simulink model "amk_eff_estimator_base"  (R2024b)
settings: Solver=FixedStepAuto  StartTime=0.0  StopTime=10.0  FixedStep=0.004  RelTol=1e-3
undefined symbols (not defined in the file): AMKData, AMKData_T100C, AMKData_T120C
settings Model: Creator=lukec  LastModifiedBy=lukec
settings OptimizationCC: DefaultParameterBehavior=Inlined  EnhancedBackFolding=on  PassReuseOutputArgsAs=Individual arguments  ZeroExternalMemoryAtStartup=off  ZeroInternalMemoryAtStartup=off  OptimizeBlockOrder=speed  DifferentSizesBufferReuse=on  OptimizationCustomize=off  EfficientTunableParamExpr=on
settings DebuggingCC: ParameterTunabilityLossMsg=error
settings HardwareCC: ProdBitPerPointer=32  ProdBitPerSizeT=32  ProdBitPerPtrDiffT=32  ProdLargestAtomicInteger=Long  ProdLargestAtomicFloat=Double  ProdWordSize=32  ProdHWDeviceType=ARM Compatible->ARM Cortex-M
settings SFSimCC: MATLABDynamicMemAlloc=off
settings RTWCC: Description=Embedded Coder  SystemTargetFile=ert.tlc  GenCodeOnly=on  PackageGeneratedCodeAndArtifacts=on  TemplateMakefile=ert_default_tmf  Toolchain=CMake  TargetLang=C++  HalideCodeGeneration=on
settings CodeAppCC: ForceParamTrailComments=on  IgnoreCustomStorageClasses=off  MaxIdLength=255  OperatorAnnotations=on  SimulinkDataObjDesc=on  SFDataObjDesc=on  InsertBlockDesc=on
settings ERTTargetCC: TargetLangStandard=C++17 (ISO)  CodeInterfacePackaging=C++ class  RootIOFormat=Structure reference  ERTCustomFileTemplate=example_file_process.tlc  ArrayContainerType=std::array

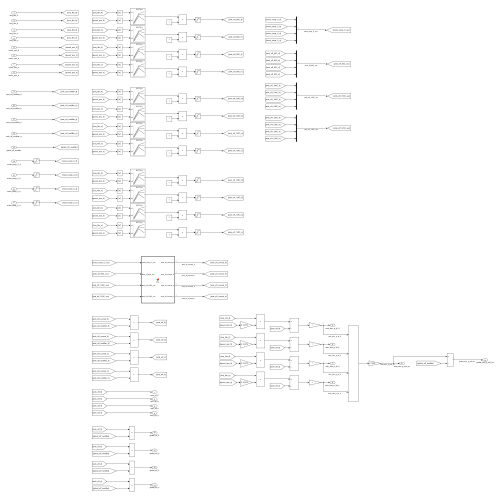
[thumbnail: Simulink's stored preview of the top-level diagram]
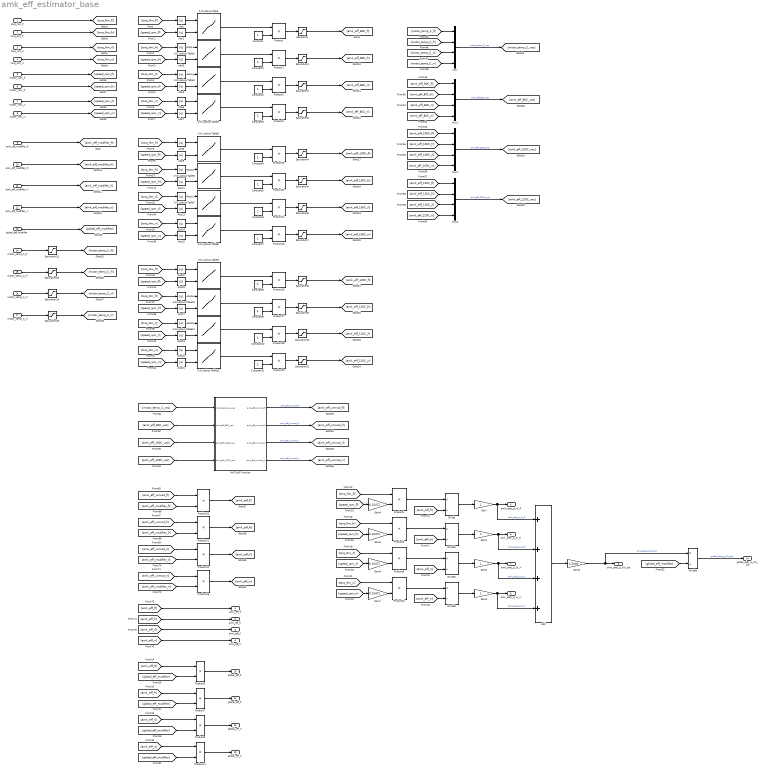
== system amk_eff_estimator_base ==
  torq_Nm_fl : Inport
  torq_Nm_fr : Inport  Port=2
  torq_Nm_rl : Inport  Port=3
  torq_Nm_rr : Inport  Port=4
  motor_rpm_fl : Inport  Port=5
  motor_rpm_fr : Inport  Port=6
  motor_rpm_rl : Inport  Port=7
  motor_rpm_rr : Inport  Port=8
  amk_eff_modifier_fl : Inport  Port=9
  amk_eff_modifier_fr : Inport  Port=10
  amk_eff_modifier_rl : Inport  Port=11
  amk_eff_modifier_rr : Inport  Port=12
  global_eff_modifier : Inport  Port=13
  motor_temp_C_fl : Inport  Port=14
  motor_temp_C_fr : Inport  Port=15
  motor_temp_C_rl : Inport  Port=16
  motor_temp_C_rr : Inport  Port=17
  2-D Lookup Table{,1..3} (4 alike) : Lookup_n-D  BreakpointsForDimension1=AMKData.torq_testpoints  BreakpointsForDimension2=AMKData.speed_testpoints  Table=AMKData.eff_zq  ExtrapMethod=Clip  UseLastTableValue=on  InternalRulePriority=Speed  RndMeth=Simplest
      settings: InputPortMap=u0,u1
  2-D Lookup Table{9..12} (4 alike) : Lookup_n-D  BreakpointsForDimension1=AMKData_T120C.torq_testpoints  BreakpointsForDimension2=AMKData_T120C.speed_testpoints  Table=AMKData_T120C.eff_zq  ExtrapMethod=Clip  UseLastTableValue=on  InternalRulePriority=Speed  RndMeth=Simplest
      settings: InputPortMap=u0,u1
  2-D Lookup Table{5..8} (4 alike) : Lookup_n-D  BreakpointsForDimension1=AMKData_T100C.torq_testpoints  BreakpointsForDimension2=AMKData_T100C.speed_testpoints  Table=AMKData_T100C.eff_zq  ExtrapMethod=Clip  UseLastTableValue=on  InternalRulePriority=Speed  RndMeth=Simplest
      settings: InputPortMap=u0,u1
  Abs{,1..23} (24 alike) : Abs  SaturateOnIntegerOverflow=off
  Add : Sum  Inputs=++++
  Constant{,1..11} (12 alike) : Constant
  Divide{,1..4} (5 alike) : Product  Inputs=*/
  Gain{,1..3} (4 alike) : Gain
  Gain{4..7} (4 alike) : Gain  Gain=0.10472
  Gain8 : Gain  Gain=1/1000
  MATLAB Function : MATLAB Function  TreatAsAtomicUnit=on
  Mux{,1..3} (4 alike) : Mux
  Product{,1..23} (24 alike) : Product
  Saturation{,1..11} (12 alike) : Saturate  UpperLimit=1  LowerLimit=0.6
  Saturation{12..15} (4 alike) : Saturate  UpperLimit=120  LowerLimit=80
  amk_eff_fl : Outport
  amk_eff_fr : Outport  Port=2
  amk_eff_rl : Outport  Port=3
  amk_eff_rr : Outport  Port=4
  amk_elec_p_W_fl : Outport  Port=5
  amk_elec_p_W_fr : Outport  Port=6
  amk_elec_p_W_rl : Outport  Port=7
  amk_elec_p_W_rr : Outport  Port=8
  amk_elec_p_kW_tot : Outport  Port=9
  global_eff_fl : Outport  Port=10
  global_eff_fr : Outport  Port=11
  global_eff_rl : Outport  Port=12
  global_eff_rr : Outport  Port=13
  global_elec_p_kW_tot : Outport  Port=14
  wires:
  torq_Nm_rl/1 -> [torq_Nm_rl]
  Constant2/1 -> Product2/2
  [speed_rpm_fl] -> Abs1/1
  Abs5/1 -> 2-D Lookup Table2/2
  motor_rpm_rr/1 -> [speed_rpm_rr]
  2-D Lookup Table/1 -> Product/1
  Product/1 -> Saturation/1
  [speed_rpm_fr] -> Abs3/1
  motor_rpm_fl/1 -> [speed_rpm_fl]
  Abs/1 -> 2-D Lookup Table/1
  Constant3/1 -> Product3/2
  2-D Lookup Table2/1 -> Product2/1
  Abs7/1 -> 2-D Lookup Table3/2
  [torq_Nm_fr] -> Abs2/1
  Abs2/1 -> 2-D Lookup Table1/1
  Constant/1 -> Product/2
  [torq_Nm_rl] -> Abs4/1
  2-D Lookup Table3/1 -> Product3/1
  torq_Nm_rr/1 -> [torq_Nm_rr]
  2-D Lookup Table1/1 -> Product1/1
  amk_eff_modifier_fl/1 -> [amk_eff_modifier_fl]
  motor_rpm_rl/1 -> [speed_rpm_rl]
  Constant1/1 -> Product1/2
  Abs1/1 -> 2-D Lookup Table/2
  torq_Nm_fl/1 -> [torq_Nm_fl]
  Abs3/1 -> 2-D Lookup Table1/2
  [torq_Nm_fl] -> Abs/1
  [speed_rpm_rl] -> Abs5/1
  Abs6/1 -> 2-D Lookup Table3/1
  motor_rpm_fr/1 -> [speed_rpm_fr]
  [speed_rpm_rr] -> Abs7/1
  Abs4/1 -> 2-D Lookup Table2/1
  [torq_Nm_rr] -> Abs6/1
  torq_Nm_fr/1 -> [torq_Nm_fr]
  [torq_Nm_fl] -> Product4/1
  [speed_rpm_fl] -> Gain4/1
  Product1/1 -> Saturation1/1
  Product2/1 -> Saturation2/1
  Product3/1 -> Saturation3/1
  Product4/1 -> Divide/1
  [amk_eff_fl] -> Divide/2
  Divide/1 -> Gain/1
  Divide1/1 -> Gain1/1
  [amk_eff_fr] -> Divide1/2
  Product6/1 -> Divide1/1
  [speed_rpm_fr] -> Gain5/1
  [torq_Nm_fr] -> Product6/1
  [torq_Nm_rl] -> Product8/1
  [speed_rpm_rl] -> Gain6/1
  Product8/1 -> Divide2/1
  [amk_eff_rl] -> Divide2/2
  Divide2/1 -> Gain2/1
  Divide3/1 -> Gain3/1
  [amk_eff_rr] -> Divide3/2
  Product10/1 -> Divide3/1
  [speed_rpm_rr] -> Gain7/1
  [torq_Nm_rr] -> Product10/1
  Gain/1 -> Add/1, amk_elec_p_W_fl/1  "amk_elec_p_W_fl"
  Gain1/1 -> Add/2, amk_elec_p_W_fr/1  "amk_elec_p_W_fr"
  Gain2/1 -> Add/3, amk_elec_p_W_rl/1  "amk_elec_p_W_rl"
  Gain3/1 -> Add/4, amk_elec_p_W_rr/1  "amk_elec_p_W_rr"
  Gain4/1 -> Product4/2
  Gain5/1 -> Product6/2
  Gain6/1 -> Product8/2
  Gain7/1 -> Product10/2
  Add/1 -> Gain8/1
  Saturation/1 -> [amk_eff_80C_fl]
  Saturation1/1 -> [amk_eff_80C_fr]
  Saturation2/1 -> [amk_eff_80C_rl]
  Saturation3/1 -> [amk_eff_80C_rr]
  amk_eff_modifier_fr/1 -> [amk_eff_modifier_fr]
  amk_eff_modifier_rl/1 -> [amk_eff_modifier_rl]
  amk_eff_modifier_rr/1 -> [amk_eff_modifier_rr]
  global_eff_modifier/1 -> [global_eff_modifier]
  [amk_eff_fl] -> Product5/1
  [global_eff_modifier] -> Product5/2
  Product5/1 -> global_eff_fl/1
  [global_eff_modifier] -> Product7/2
  [amk_eff_fr] -> Product7/1
  Product7/1 -> global_eff_fr/1
  [global_eff_modifier] -> Product9/2
  [amk_eff_rl] -> Product9/1
  Product9/1 -> global_eff_rl/1
  [global_eff_modifier] -> Product11/2
  [amk_eff_rr] -> Product11/1
  Product11/1 -> global_eff_rr/1
  [global_eff_modifier] -> Divide4/2
  Divide4/1 -> global_elec_p_kW_tot/1  "global_elec_p_kW_tot"
  Gain8/1 -> Divide4/1, amk_elec_p_kW_tot/1  "amk_elec_p_kW_tot"
  Product15/1 -> Saturation7/1
  Product14/1 -> Saturation6/1
  Product13/1 -> Saturation5/1
  [torq_Nm_rr] -> Abs14/1
  Abs12/1 -> 2-D Lookup Table7/1
  [speed_rpm_rr] -> Abs15/1
  Abs14/1 -> 2-D Lookup Table8/1
  [speed_rpm_rl] -> Abs13/1
  [torq_Nm_fl] -> Abs8/1
  Abs11/1 -> 2-D Lookup Table6/2
  Abs9/1 -> 2-D Lookup Table5/2
  Constant5/1 -> Product13/2
  2-D Lookup Table6/1 -> Product13/1
  2-D Lookup Table8/1 -> Product15/1
  [torq_Nm_rl] -> Abs12/1
  Constant4/1 -> Product12/2
  Abs10/1 -> 2-D Lookup Table6/1
  [torq_Nm_fr] -> Abs10/1
  Abs15/1 -> 2-D Lookup Table8/2
  2-D Lookup Table7/1 -> Product14/1
  Constant7/1 -> Product15/2
  Abs8/1 -> 2-D Lookup Table5/1
  [speed_rpm_fr] -> Abs11/1
  Product12/1 -> Saturation4/1
  2-D Lookup Table5/1 -> Product12/1
  Abs13/1 -> 2-D Lookup Table7/2
  [speed_rpm_fl] -> Abs9/1
  Constant6/1 -> Product14/2
  Constant10/1 -> Product18/2
  [speed_rpm_fl] -> Abs23/1
  Abs19/1 -> 2-D Lookup Table11/2
  2-D Lookup Table9/1 -> Product16/1
  Product16/1 -> Saturation8/1
  [speed_rpm_fr] -> Abs17/1
  Abs22/1 -> 2-D Lookup Table9/1
  Constant11/1 -> Product19/2
  2-D Lookup Table11/1 -> Product18/1
  Abs21/1 -> 2-D Lookup Table12/2
  [torq_Nm_fr] -> Abs16/1
  Abs16/1 -> 2-D Lookup Table10/1
  Constant8/1 -> Product16/2
  [torq_Nm_rl] -> Abs18/1
  2-D Lookup Table12/1 -> Product19/1
  2-D Lookup Table10/1 -> Product17/1
  Constant9/1 -> Product17/2
  Abs23/1 -> 2-D Lookup Table9/2
  Abs17/1 -> 2-D Lookup Table10/2
  [torq_Nm_fl] -> Abs22/1
  [speed_rpm_rl] -> Abs19/1
  Abs20/1 -> 2-D Lookup Table12/1
  [speed_rpm_rr] -> Abs21/1
  Abs18/1 -> 2-D Lookup Table11/1
  [torq_Nm_rr] -> Abs20/1
  Product17/1 -> Saturation9/1
  Product18/1 -> Saturation10/1
  Product19/1 -> Saturation11/1
  Saturation4/1 -> [amk_eff_100C_fl]
  Saturation5/1 -> [amk_eff_100C_fr]
  Saturation6/1 -> [amk_eff_100C_rl]
  Saturation7/1 -> [amk_eff_100C_rr]
  Saturation8/1 -> [amk_eff_120C_fl]
  Saturation9/1 -> [amk_eff_120C_fr]
  Saturation10/1 -> [amk_eff_120C_rl]
  Saturation11/1 -> [amk_eff_120C_rr]
  motor_temp_C_fl/1 -> Saturation12/1
  motor_temp_C_fr/1 -> Saturation13/1
  motor_temp_C_rl/1 -> Saturation14/1
  motor_temp_C_rr/1 -> Saturation15/1
  Saturation12/1 -> [motor_temp_C_fl]
  Saturation13/1 -> [motor_temp_C_fr]
  Saturation14/1 -> [motor_temp_C_rl]
  Saturation15/1 -> [motor_temp_C_rr]
  [motor_temp_C_fl] -> Mux/1
  [motor_temp_C_fr] -> Mux/2
  [motor_temp_C_rl] -> Mux/3
  [motor_temp_C_rr] -> Mux/4
  Mux/1 -> [motor_temp_C_vec]  "motor_temp_C_vec"
  [amk_eff_80C_fl] -> Mux1/1
  [amk_eff_80C_fr] -> Mux1/2
  [amk_eff_80C_rl] -> Mux1/3
  [amk_eff_80C_rr] -> Mux1/4
  Mux1/1 -> [amk_eff_80C_vec]  "amk_eff_80C_vec"
  Mux2/1 -> [amk_eff_100C_vec]  "amk_eff_100C_vec"
  [amk_eff_100C_rr] -> Mux2/4
  [amk_eff_100C_rl] -> Mux2/3
  [amk_eff_100C_fr] -> Mux2/2
  [amk_eff_100C_fl] -> Mux2/1
  [amk_eff_120C_fl] -> Mux3/1
  [amk_eff_120C_fr] -> Mux3/2
  [amk_eff_120C_rl] -> Mux3/3
  [amk_eff_120C_rr] -> Mux3/4
  Mux3/1 -> [amk_eff_120C_vec]  "amk_eff_120C_vec"
  [motor_temp_C_vec] -> MATLAB Function/1(motor_temp_C_vec)
  [amk_eff_80C_vec] -> MATLAB Function/2(amk_eff_80C_vec)
  [amk_eff_100C_vec] -> MATLAB Function/3(amk_eff_100C_vec)
  [amk_eff_120C_vec] -> MATLAB Function/4(amk_eff_120C_vec)
  MATLAB Function/1(amk_eff_unmod_fl) -> [amk_eff_unmod_fl]  "amk_eff_unmod_fl"
  MATLAB Function/2(amk_eff_unmod_fr) -> [amk_eff_unmod_fr]  "amk_eff_unmod_fr"
  MATLAB Function/3(amk_eff_unmod_rl) -> [amk_eff_unmod_rl]  "amk_eff_unmod_rl"
  MATLAB Function/4(amk_eff_unmod_rr) -> [amk_eff_unmod_rr]  "amk_eff_unmod_rr"
  [amk_eff_unmod_fl] -> Product20/1
  [amk_eff_modifier_fl] -> Product20/2
  Product20/1 -> [amk_eff_fl]
  Product21/1 -> [amk_eff_fr]
  [amk_eff_modifier_fr] -> Product21/2
  [amk_eff_unmod_fr] -> Product21/1
  [amk_eff_unmod_rl] -> Product22/1
  [amk_eff_modifier_rl] -> Product22/2
  Product22/1 -> [amk_eff_rl]
  Product23/1 -> [amk_eff_rr]
  [amk_eff_modifier_rr] -> Product23/2
  [amk_eff_unmod_rr] -> Product23/1
  [amk_eff_fl] -> amk_eff_fl/1
  [amk_eff_fr] -> amk_eff_fr/1
  [amk_eff_rl] -> amk_eff_rl/1
  [amk_eff_rr] -> amk_eff_rr/1

== matlab function amk_eff_estimator_base/MATLAB Function ==
  data: motor_temp_C_vec input; amk_eff_unmod_fl output; amk_eff_80C_vec input; amk_eff_100C_vec input; amk_eff_120C_vec input; amk_eff_unmod_fr output; amk_eff_unmod_rl output; amk_eff_unmod_rr output
function [amk_eff_unmod_fl, amk_eff_unmod_fr, amk_eff_unmod_rl, amk_eff_unmod_rr]  = fcn(motor_temp_C_vec, amk_eff_80C_vec, amk_eff_100C_vec, amk_eff_120C_vec)

amk_eff_vec = [1; 1; 1; 1];

for i = 1:4
    temp_C = motor_temp_C_vec(i);
    eff_80C = amk_eff_80C_vec(i);
    eff_100C = amk_eff_100C_vec(i);
    eff_120C = amk_eff_120C_vec(i);

    amk_eff_vec(i) = interp1([80, 100, 120], [eff_80C, eff_100C, eff_120C], temp_C);
end

amk_eff_unmod_fl = amk_eff_vec(1);
amk_eff_unmod_fr = amk_eff_vec(2);
amk_eff_unmod_rl = amk_eff_vec(3);
amk_eff_unmod_rr = amk_eff_vec(4);
